simulink model "controller"  (R2023b)
settings: Solver=FixedStepDiscrete  StartTime=0.0  StopTime=inf  FixedStep=1/100  RelTol=1e-3
model workspace (MAT data in the model file):
  dt = Simulink.Parameter
  dt.Value = 0.0025
  dt.DataType = 'auto'
  dt.Complexity = 'real'
  dt.Dimensions = [1 1]
libraries: slpidlib x3
settings Model: Creator=asd  LastModifiedBy=asd
settings SolverCC: InsertRTBMode=Always
settings DataIOCC: ExternalInput=dt  InitialState=[dt]
settings OptimizationCC: DefaultParameterBehavior=Inlined  DefaultUnderspecifiedDataType=single  EnhancedBackFolding=on  PassReuseOutputArgsAs=Individual arguments  ZeroExternalMemoryAtStartup=off  ZeroInternalMemoryAtStartup=off  OptimizeBlockOrder=speed  DifferentSizesBufferReuse=on  OptimizationCustomize=off  LabelGuidedReuse=on  EfficientTunableParamExpr=on
settings DebuggingCC: ParameterTunabilityLossMsg=error
settings HardwareCC: ProdBitPerPointer=32  ProdBitPerSizeT=32  ProdBitPerPtrDiffT=32  ProdLargestAtomicInteger=Long  ProdLargestAtomicFloat=Double  ProdWordSize=32  ProdHWDeviceType=ARM Compatible->ARM Cortex-M
settings SFSimCC: MATLABDynamicMemAlloc=off
settings RTWCC: Description=Embedded Coder  SystemTargetFile=ert.tlc  GenCodeOnly=on  TemplateMakefile=ert_default_tmf  CustomSourceCode="#pragma GCC diagnostic ignored \"-Wfloat-equal\""  DataTypeReplacement=CDataTypesFixedWidth  TargetLang=C++
settings CodeAppCC: ForceParamTrailComments=on  IgnoreCustomStorageClasses=off  OperatorAnnotations=on  SimulinkDataObjDesc=on  SFDataObjDesc=on  InsertBlockDesc=on
settings ERTTargetCC: TargetLangStandard=C++11 (ISO)  GenerateSampleERTMain=on  CombineSignalStateStructs=on  GroupInternalDataByFunction=on  CodeInterfacePackaging=C++ class  SupportComplex=off  DSAsUniqueAccess=on  ExtModeTransport=2  ExtModeStaticAlloc=on  ExtModeMaxTrigDuration=1000000  ExtModeMexFile=ext_xcp  ExtModeIntrfLevel=Level2 - Open  RootIOFormat=Structure reference  ERTCustomFileTemplate=example_file_process.tlc  MaxIdInt64=INT64_MAX  MinIdInt64=INT64_MIN  MaxIdUint64=UINT64_MAX  MaxIdInt32=INT32_MAX  MinIdInt32=INT32_MIN  MaxIdUint32=UINT32_MAX  MaxIdInt16=INT16_MAX  MinIdInt16=INT16_MIN  MaxIdUint16=UINT16_MAX  MaxIdInt8=INT8_MAX  MinIdInt8=INT8_MIN  MaxIdUint8=UINT8_MAX

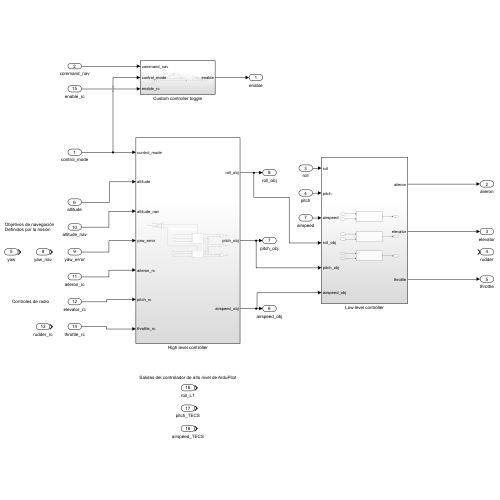
[thumbnail: Simulink's stored preview of the top-level diagram]
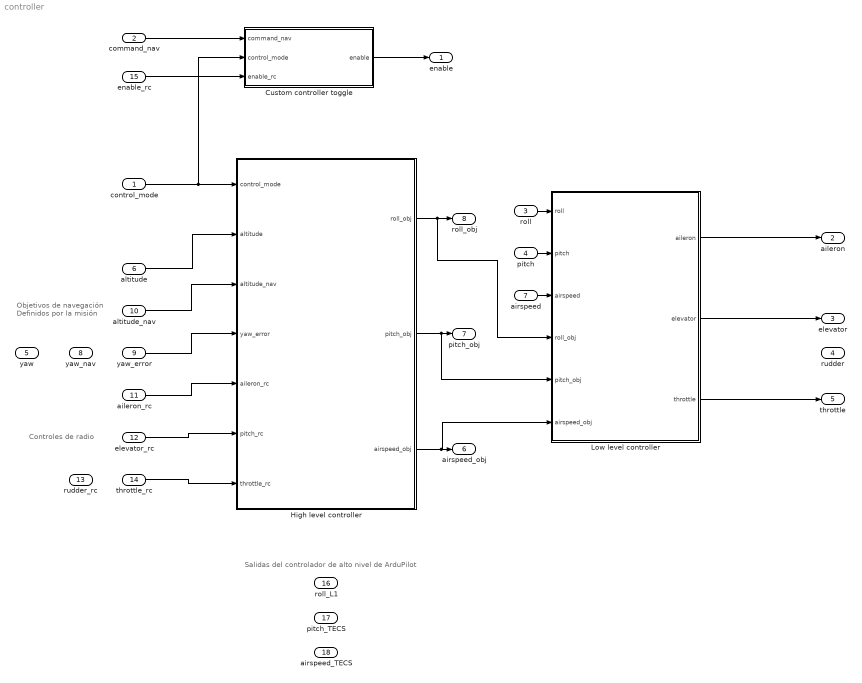
== system controller ==
  note: Controles de radio
  note: Objetivos de navegación
      | Definidos por la misión
  note: Salidas del controlador de alto nivel de ArduPilot
  control_mode : Inport  OutDataTypeStr=single
  command_nav : Inport  Port=2
  roll : Inport  Port=3
  pitch : Inport  Port=4
  yaw : Inport  Port=5
  altitude : Inport  Port=6
  airspeed : Inport  Port=7  OutDataTypeStr=single
  yaw_nav : Inport  Port=8
  yaw_error : Inport  Port=9
  altitude_nav : Inport  Port=10
  aileron_rc : Inport  Port=11
  elevator_rc : Inport  Port=12
  rudder_rc : Inport  Port=13
  throttle_rc : Inport  Port=14  OutDataTypeStr=single
  enable_rc : Inport  Port=15  OutDataTypeStr=boolean
  roll_L1 : Inport  Port=16
  pitch_TECS : Inport  Port=17
  airspeed_TECS : Inport  Port=18
  Custom controller toggle : Subsystem
  High level controller : Subsystem
  Low level controller : Subsystem
  enable : Outport  OutDataTypeStr=boolean
  aileron : Outport  Port=2
  elevator : Outport  Port=3
  rudder : Outport  Port=4
  throttle : Outport  Port=5  OutDataTypeStr=single
  airspeed_obj : Outport  Port=6  OutDataTypeStr=single
  pitch_obj : Outport  Port=7
  roll_obj : Outport  Port=8
  wires:
  control_mode/1 -> Custom controller toggle/2(control_mode), High level controller/1(control_mode)
  altitude/1 -> High level controller/2(altitude)
  altitude_nav/1 -> High level controller/3(altitude_nav)
  yaw_error/1 -> High level controller/4(yaw_error)
  aileron_rc/1 -> High level controller/5(aileron_rc)
  elevator_rc/1 -> High level controller/6(pitch_rc)
  throttle_rc/1 -> High level controller/7(throttle_rc)
  High level controller/1(roll_obj) -> roll_obj/1, Low level controller/4(roll_obj)
  roll/1 -> Low level controller/1(roll)
  High level controller/2(pitch_obj) -> pitch_obj/1, Low level controller/5(pitch_obj)
  pitch/1 -> Low level controller/2(pitch)
  High level controller/3(airspeed_obj) -> Low level controller/6(airspeed_obj), airspeed_obj/1
  Low level controller/1(aileron) -> aileron/1
  Low level controller/2(elevator) -> elevator/1
  Low level controller/3(throttle) -> throttle/1
  airspeed/1 -> Low level controller/3(airspeed)
  command_nav/1 -> Custom controller toggle/1(command_nav)
  Custom controller toggle/1(enable) -> enable/1
  enable_rc/1 -> Custom controller toggle/3(enable_rc)

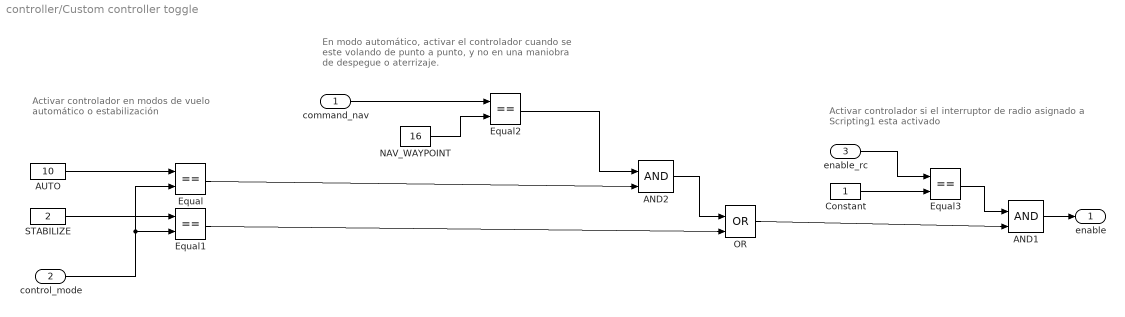
== system controller/Custom controller toggle ==
  note: Activar controlador si el interruptor de radio asignado
      | a Scripting1 esta activado
  note: En modo automático, activar el controlador cuando
      | se este volando de punto a punto, y no en una
      | maniobra de despegue o aterrizaje.
  note: Activar controlador en modos de vuelo
      | automático o estabilización
  command_nav : Inport
  control_mode : Inport  Port=2
  enable_rc : Inport  Port=3  OutDataTypeStr=boolean
  AND1 : Logic  IconShape=distinctive  AllPortsSameDT=off  OutDataTypeStr=boolean
  AND2 : Logic  IconShape=distinctive  AllPortsSameDT=off  OutDataTypeStr=boolean
  AUTO : Constant  Value=10  OutDataTypeStr=single
  Constant : Constant  OutDataTypeStr=boolean
  Equal{,1..3} (4 alike) : RelationalOperator  Operator===  OutDataTypeStr=boolean  RndMeth=Simplest  InputSameDT=off
  NAV_WAYPOINT : Constant  Value=16  OutDataTypeStr=single
  OR : Logic  Operator=OR  IconShape=distinctive  AllPortsSameDT=off  OutDataTypeStr=boolean
  STABILIZE : Constant  Value=2  OutDataTypeStr=single
  enable : Outport
  wires:
  Equal1/1 -> OR/2
  control_mode/1 -> Equal/2, Equal1/2
  STABILIZE/1 -> Equal1/1
  AUTO/1 -> Equal/1
  NAV_WAYPOINT/1 -> Equal2/2
  command_nav/1 -> Equal2/1
  AND1/1 -> enable/1
  Constant/1 -> Equal3/2
  enable_rc/1 -> Equal3/1
  Equal3/1 -> AND1/1
  Equal2/1 -> AND2/1
  Equal/1 -> AND2/2
  AND2/1 -> OR/1
  OR/1 -> AND1/2

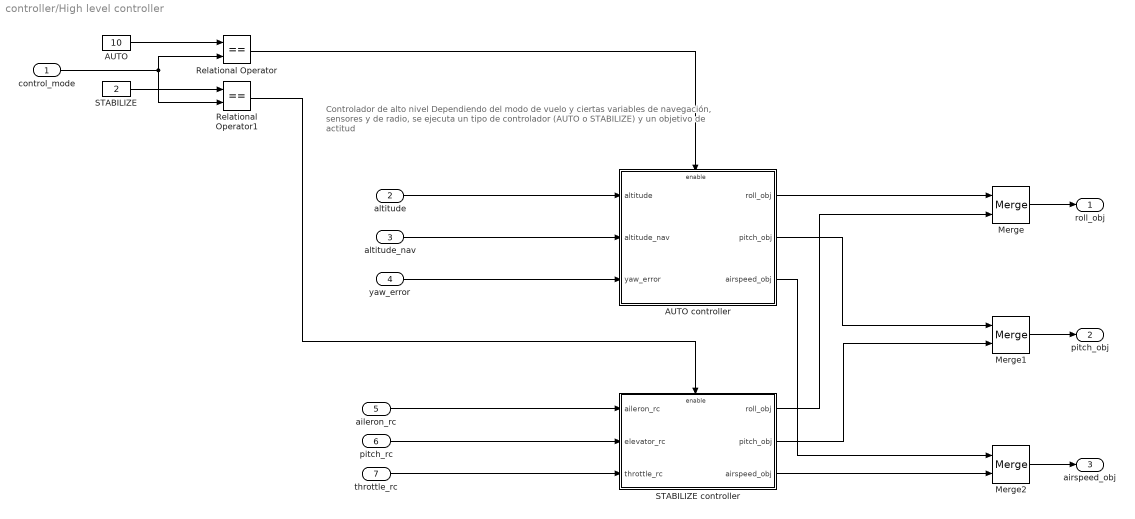
== system controller/High level controller ==
  note: Controlador de alto nivel
      | Dependiendo del modo de vuelo y ciertas variables de navegación, sensores y de radio,
      | se ejecuta un tipo de controlador (AUTO o STABILIZE) y un objetivo de actitud
  control_mode : Inport
  altitude : Inport  Port=2
  altitude_nav : Inport  Port=3
  yaw_error : Inport  Port=4
  aileron_rc : Inport  Port=5
  pitch_rc : Inport  Port=6
  throttle_rc : Inport  Port=7
  AUTO : Constant  Value=10
  AUTO controller : Subsystem
  Merge : Merge
  Merge1 : Merge
  Merge2 : Merge
  Relational Operator : RelationalOperator  Operator===  OutDataTypeStr=boolean  RndMeth=Simplest  InputSameDT=off
  Relational Operator1 : RelationalOperator  Operator===  OutDataTypeStr=boolean  RndMeth=Simplest  InputSameDT=off
  STABILIZE : Constant  Value=2
  STABILIZE controller : Subsystem
  roll_obj : Outport
  pitch_obj : Outport  Port=2
  airspeed_obj : Outport  Port=3
  wires:
  AUTO/1 -> Relational Operator/1
  Merge2/1 -> airspeed_obj/1
  STABILIZE/1 -> Relational Operator1/1
  control_mode/1 -> Relational Operator1/2, Relational Operator/2
  Relational Operator/1 -> AUTO controller/Enable
  pitch_rc/1 -> STABILIZE controller/2(elevator_rc)
  Relational Operator1/1 -> STABILIZE controller/Enable
  altitude_nav/1 -> AUTO controller/2(altitude_nav)
  yaw_error/1 -> AUTO controller/3(yaw_error)
  altitude/1 -> AUTO controller/1(altitude)
  Merge/1 -> roll_obj/1
  throttle_rc/1 -> STABILIZE controller/3(throttle_rc)
  aileron_rc/1 -> STABILIZE controller/1(aileron_rc)
  Merge1/1 -> pitch_obj/1
  AUTO controller/1(roll_obj) -> Merge/1
  STABILIZE controller/1(roll_obj) -> Merge/2
  AUTO controller/2(pitch_obj) -> Merge1/1
  STABILIZE controller/2(pitch_obj) -> Merge1/2
  STABILIZE controller/3(airspeed_obj) -> Merge2/2
  AUTO controller/3(airspeed_obj) -> Merge2/1

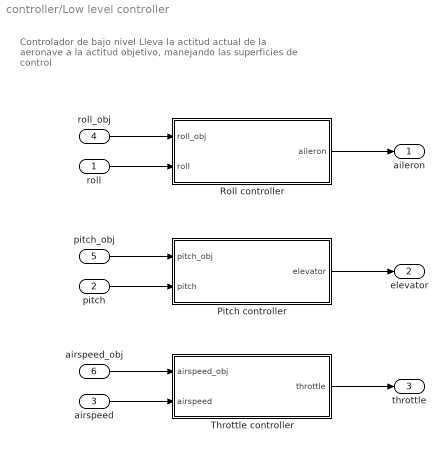
== system controller/Low level controller ==
  note: Controlador de bajo nivel
      | Lleva la actitud actual de la aeronave a la actitud objetivo,
      | manejando las superficies de control
  roll : Inport
  pitch : Inport  Port=2
  airspeed : Inport  Port=3
  roll_obj : Inport  Port=4
  pitch_obj : Inport  Port=5
  airspeed_obj : Inport  Port=6
  Pitch controller : Subsystem
  Roll controller : Subsystem
  Throttle controller : Subsystem
  aileron : Outport
  elevator : Outport  Port=2
  throttle : Outport  Port=3
  wires:
  Pitch controller/1(elevator) -> elevator/1
  Throttle controller/1(throttle) -> throttle/1
  roll/1 -> Roll controller/2(roll)
  pitch/1 -> Pitch controller/2(pitch)
  pitch_obj/1 -> Pitch controller/1(pitch_obj)
  Roll controller/1(aileron) -> aileron/1
  roll_obj/1 -> Roll controller/1(roll_obj)
  airspeed_obj/1 -> Throttle controller/1(airspeed_obj)
  airspeed/1 -> Throttle controller/2(airspeed)

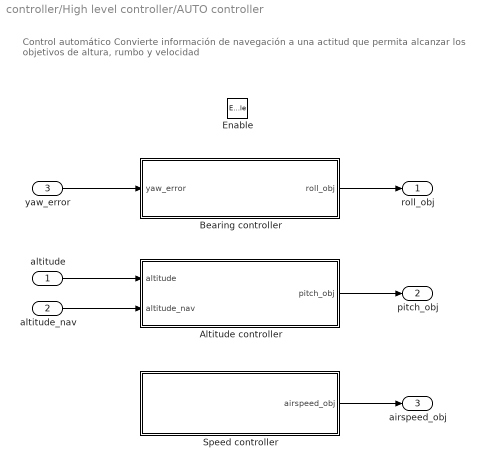
== system controller/High level controller/AUTO controller ==
  note: Control automático
      | Convierte información de navegación a una actitud que permita alcanzar los objetivos de altura, rumbo y velocidad
  altitude : Inport
  altitude_nav : Inport  Port=2
  yaw_error : Inport  Port=3
  Enable : EnablePort
  Altitude controller : Subsystem
  Bearing controller : Subsystem
  Speed controller : Subsystem
  roll_obj : Outport
  pitch_obj : Outport  Port=2
  airspeed_obj : Outport  Port=3
  wires:
  yaw_error/1 -> Bearing controller/1(yaw_error)
  altitude_nav/1 -> Altitude controller/2(altitude_nav)
  altitude/1 -> Altitude controller/1(altitude)
  Speed controller/1(airspeed_obj) -> airspeed_obj/1
  Bearing controller/1(roll_obj) -> roll_obj/1
  Altitude controller/1(pitch_obj) -> pitch_obj/1

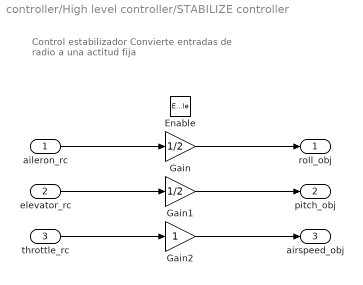
== system controller/High level controller/STABILIZE controller ==
  note: Control estabilizador
      | Convierte entradas de radio a una actitud fija
  aileron_rc : Inport
  elevator_rc : Inport  Port=2
  throttle_rc : Inport  Port=3
  Enable : EnablePort
  Gain : Gain  Gain=1/2
  Gain1 : Gain  Gain=1/2
  Gain2 : Gain
  roll_obj : Outport
  pitch_obj : Outport  Port=2
  airspeed_obj : Outport  Port=3
  wires:
  elevator_rc/1 -> Gain1/1
  aileron_rc/1 -> Gain/1
  Gain2/1 -> airspeed_obj/1
  throttle_rc/1 -> Gain2/1
  Gain1/1 -> pitch_obj/1
  Gain/1 -> roll_obj/1

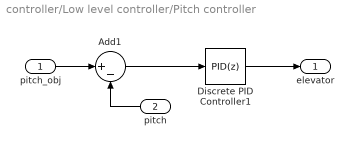
== system controller/Low level controller/Pitch controller ==
  pitch_obj : Inport
  pitch : Inport  Port=2
  Add1 : Sum  Inputs=|+-
  Discrete PID Controller1 : slpidlib/PID Controller  Controller=PID  Form=Parallel  TimeDomain=Discrete-time  UseExternalTs=off  SampleTime=-1  IntegratorMethod=Forward Euler  FilterMethod=Forward Euler  ControllerParametersSource=internal  P=1  I=0.1  UseKiTs=off  D=0.1  N=100  UseFilter=on  TunerSelectOption=Transfer Function Based (PID Tuner App)  InitialConditionSource=internal  InitialConditionForIntegrator=0  InitialConditionForFilter=0  DifferentiatorICPrevScaledInput=0  ExternalReset=none  TrackingMode=off  Kt=1  LimitOutput=off  SatLimitsSource=internal  UpperSaturationLimit=inf  LowerSaturationLimit=-inf  LinearizeAsGain=off  AntiWindupMode=none  Kb=1  LimitIntegrator=off  UpperIntegratorSaturationLimit=inf  LowerIntegratorSaturationLimit=-inf  POutMin=[]  POutMax=[]  IOutMin=[]  IOutMax=[]  DOutMin=[]  DOutMax=[]  NOutMin=[]  NOutMax=[]  SumOutMin=[]  SumOutMax=[]  SaturationOutMin=[]  SaturationOutMax=[]  PParamMin=[]  PParamMax=[]  IParamMin=[]  IParamMax=[]  DParamMin=[]  DParamMax=[]  NParamMin=[]  NParamMax=[]  KbParamMin=[]  KbParamMax=[]  KtParamMin=[]  KtParamMax=[]  KbOutMin=[]  KbOutMax=[]  KtOutMin=[]  KtOutMax=[]  IntegratorOutMin=[]  IntegratorOutMax=[]  FilterOutMin=[]  FilterOutMax=[]  SumI1OutMin=[]  SumI1OutMax=[]  SumI2OutMin=[]  SumI2OutMax=[]  SumI3OutMin=[]  SumI3OutMax=[]  SumI4OutMin=[]  SumI4OutMax=[]  SumDOutMin=[]  SumDOutMax=[]  DifferentiatorOutMin=[]  DifferentiatorOutMax=[]  FilterDiffOutCoefMin=[]  FilterDiffOutCoefMax=[]  ReciprocalOutMin=[]  ReciprocalOutMax=[]  SumDenOutMin=[]  SumDenOutMax=[]  SumNumOutMin=[]  SumNumOutMax=[]  DivideOutMin=[]  DivideOutMax=[]  UdiffTsProdOutMin=[]  UdiffTsProdOutMax=[]  NTsProdOutMin=[]  NTsProdOutMax=[]  UintegralTsProdOutMin=[]  UintegralTsProdOutMax=[]  UngainTsProdOutMin=[]  UngainTsProdOutMax=[]  ClampingZeroOutDataTypeStr=Inherit: Inherit via back propagation  ClampingZeroOutMin=[]  ClampingZeroOutMax=[]  FilterDenConstantOutDataTypeStr=Inherit: Inherit via back propagation  FilterDenConstantOutMin=[]  FilterDenConstantOutMax=[]  PCopyOutDataTypeStr=Inherit: Inherit via back propagation  PCopyOutMin=[]  PCopyOutMax=[]  NCopyOutDataTypeStr=Inherit: Inherit via back propagation  NCopyOutMin=[]  NCopyOutMax=[]  IntegratorContinuousStateAttributes=''  IntegratorStateMustResolveToSignalObject=off  IntegratorRTWStateStorageClass=Auto  FilterContinuousStateAttributes=''  FilterStateMustResolveToSignalObject=off  FilterRTWStateStorageClass=Auto  ParallelPVariant=InternalParameters  IdealPVariant=Disabled  IVariant=InternalParameters  DVariant=InternalParameters  IntegratorVariant=Discrete  SatVariant=Disabled  AWVariant=Passthrough  PCopyVariant=Disabled  TRVariant=Disabled  FdbkBlocksVariant=Forward  IdealPFdbkVariant=Disabled  SatFdbkVariant=Disabled  DerivativeFilterVariant=ForwardEulerFilter  NVariant=InternalParameters  NCopyVariant=Disabled  FilterICVariant=InternalICsFilter  IntegratorICVariant=InternalICs  ExternalResetVariant=Disabled  TRSumVariant=Passthrough  SumFdbkVariant=Disabled  SumVariant=Sum_PID  TsampFilterVariant=InternalTs  TsampNgainVariant=Passthrough  TsampIntegralVariant=Disabled_SignalSpec  ExternalSaturationOutDataTypeStr=Inherit: Same as second input
      settings: LibrarySourceBlock=simulink/Discrete/Discrete PID Controller
  elevator : Outport
  wires:
  pitch_obj/1 -> Add1/1
  Add1/1 -> Discrete PID Controller1/1
  Discrete PID Controller1/1 -> elevator/1
  pitch/1 -> Add1/2

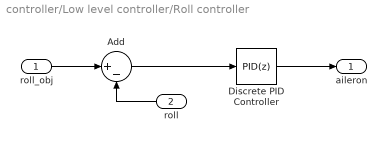
== system controller/Low level controller/Roll controller ==
  roll_obj : Inport
  roll : Inport  Port=2
  Add : Sum  Inputs=|+-
  Discrete PID Controller : slpidlib/PID Controller  Controller=PID  Form=Parallel  TimeDomain=Discrete-time  UseExternalTs=off  SampleTime=-1  IntegratorMethod=Forward Euler  FilterMethod=Forward Euler  ControllerParametersSource=internal  P=1  I=0  UseKiTs=off  D=0.5  N=100  UseFilter=on  TunerSelectOption=Transfer Function Based (PID Tuner App)  InitialConditionSource=internal  InitialConditionForIntegrator=0  InitialConditionForFilter=0  DifferentiatorICPrevScaledInput=0  ExternalReset=none  TrackingMode=off  Kt=1  LimitOutput=off  SatLimitsSource=internal  UpperSaturationLimit=inf  LowerSaturationLimit=-inf  LinearizeAsGain=off  AntiWindupMode=none  Kb=1  LimitIntegrator=off  UpperIntegratorSaturationLimit=inf  LowerIntegratorSaturationLimit=-inf  POutMin=[]  POutMax=[]  IOutMin=[]  IOutMax=[]  DOutMin=[]  DOutMax=[]  NOutMin=[]  NOutMax=[]  SumOutMin=[]  SumOutMax=[]  SaturationOutMin=[]  SaturationOutMax=[]  PParamMin=[]  PParamMax=[]  IParamMin=[]  IParamMax=[]  DParamMin=[]  DParamMax=[]  NParamMin=[]  NParamMax=[]  KbParamMin=[]  KbParamMax=[]  KtParamMin=[]  KtParamMax=[]  KbOutMin=[]  KbOutMax=[]  KtOutMin=[]  KtOutMax=[]  IntegratorOutMin=[]  IntegratorOutMax=[]  FilterOutMin=[]  FilterOutMax=[]  SumI1OutMin=[]  SumI1OutMax=[]  SumI2OutMin=[]  SumI2OutMax=[]  SumI3OutMin=[]  SumI3OutMax=[]  SumI4OutMin=[]  SumI4OutMax=[]  SumDOutMin=[]  SumDOutMax=[]  DifferentiatorOutMin=[]  DifferentiatorOutMax=[]  FilterDiffOutCoefMin=[]  FilterDiffOutCoefMax=[]  ReciprocalOutMin=[]  ReciprocalOutMax=[]  SumDenOutMin=[]  SumDenOutMax=[]  SumNumOutMin=[]  SumNumOutMax=[]  DivideOutMin=[]  DivideOutMax=[]  UdiffTsProdOutMin=[]  UdiffTsProdOutMax=[]  NTsProdOutMin=[]  NTsProdOutMax=[]  UintegralTsProdOutMin=[]  UintegralTsProdOutMax=[]  UngainTsProdOutMin=[]  UngainTsProdOutMax=[]  ClampingZeroOutDataTypeStr=Inherit: Inherit via back propagation  ClampingZeroOutMin=[]  ClampingZeroOutMax=[]  FilterDenConstantOutDataTypeStr=Inherit: Inherit via back propagation  FilterDenConstantOutMin=[]  FilterDenConstantOutMax=[]  PCopyOutDataTypeStr=Inherit: Inherit via back propagation  PCopyOutMin=[]  PCopyOutMax=[]  NCopyOutDataTypeStr=Inherit: Inherit via back propagation  NCopyOutMin=[]  NCopyOutMax=[]  IntegratorContinuousStateAttributes=''  IntegratorStateMustResolveToSignalObject=off  IntegratorRTWStateStorageClass=Auto  FilterContinuousStateAttributes=''  FilterStateMustResolveToSignalObject=off  FilterRTWStateStorageClass=Auto  ParallelPVariant=InternalParameters  IdealPVariant=Disabled  IVariant=InternalParameters  DVariant=InternalParameters  IntegratorVariant=Discrete  SatVariant=Disabled  AWVariant=Passthrough  PCopyVariant=Disabled  TRVariant=Disabled  FdbkBlocksVariant=Forward  IdealPFdbkVariant=Disabled  SatFdbkVariant=Disabled  DerivativeFilterVariant=ForwardEulerFilter  NVariant=InternalParameters  NCopyVariant=Disabled  FilterICVariant=InternalICsFilter  IntegratorICVariant=InternalICs  ExternalResetVariant=Disabled  TRSumVariant=Passthrough  SumFdbkVariant=Disabled  SumVariant=Sum_PID  TsampFilterVariant=InternalTs  TsampNgainVariant=Passthrough  TsampIntegralVariant=Disabled_SignalSpec  ExternalSaturationOutDataTypeStr=Inherit: Same as second input
      settings: LibrarySourceBlock=simulink/Discrete/Discrete PID Controller
  aileron : Outport
  wires:
  Add/1 -> Discrete PID Controller/1
  roll/1 -> Add/2
  Discrete PID Controller/1 -> aileron/1
  roll_obj/1 -> Add/1

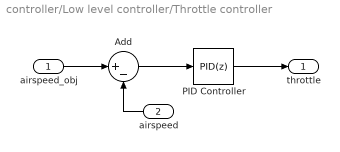
== system controller/Low level controller/Throttle controller ==
  airspeed_obj : Inport
  airspeed : Inport  Port=2
  Add : Sum  Inputs=|+-
  PID Controller : slpidlib/PID Controller  Controller=PID  Form=Parallel  TimeDomain=Discrete-time  UseExternalTs=off  SampleTime=-1  IntegratorMethod=Forward Euler  FilterMethod=Forward Euler  ControllerParametersSource=internal  P=5  I=1  UseKiTs=off  D=1  N=100  UseFilter=on  TunerSelectOption=Transfer Function Based (PID Tuner App)  InitialConditionSource=internal  InitialConditionForIntegrator=0  InitialConditionForFilter=0  DifferentiatorICPrevScaledInput=0  ExternalReset=none  TrackingMode=off  Kt=1  LimitOutput=off  SatLimitsSource=internal  UpperSaturationLimit=inf  LowerSaturationLimit=-inf  LinearizeAsGain=on  AntiWindupMode=none  Kb=1  LimitIntegrator=off  UpperIntegratorSaturationLimit=inf  LowerIntegratorSaturationLimit=-inf  POutMin=[]  POutMax=[]  IOutMin=[]  IOutMax=[]  DOutMin=[]  DOutMax=[]  NOutMin=[]  NOutMax=[]  SumOutMin=[]  SumOutMax=[]  SaturationOutMin=[]  SaturationOutMax=[]  PParamMin=[]  PParamMax=[]  IParamMin=[]  IParamMax=[]  DParamMin=[]  DParamMax=[]  NParamMin=[]  NParamMax=[]  KbParamMin=[]  KbParamMax=[]  KtParamMin=[]  KtParamMax=[]  KbOutMin=[]  KbOutMax=[]  KtOutMin=[]  KtOutMax=[]  IntegratorOutMin=[]  IntegratorOutMax=[]  FilterOutMin=[]  FilterOutMax=[]  SumI1OutMin=[]  SumI1OutMax=[]  SumI2OutMin=[]  SumI2OutMax=[]  SumI3OutMin=[]  SumI3OutMax=[]  SumI4OutMin=[]  SumI4OutMax=[]  SumDOutMin=[]  SumDOutMax=[]  DifferentiatorOutMin=[]  DifferentiatorOutMax=[]  FilterDiffOutCoefMin=[]  FilterDiffOutCoefMax=[]  ReciprocalOutMin=[]  ReciprocalOutMax=[]  SumDenOutMin=[]  SumDenOutMax=[]  SumNumOutMin=[]  SumNumOutMax=[]  DivideOutMin=[]  DivideOutMax=[]  UdiffTsProdOutMin=[]  UdiffTsProdOutMax=[]  NTsProdOutMin=[]  NTsProdOutMax=[]  UintegralTsProdOutMin=[]  UintegralTsProdOutMax=[]  UngainTsProdOutMin=[]  UngainTsProdOutMax=[]  ClampingZeroOutDataTypeStr=Inherit: Inherit via back propagation  ClampingZeroOutMin=[]  ClampingZeroOutMax=[]  FilterDenConstantOutDataTypeStr=Inherit: Inherit via back propagation  FilterDenConstantOutMin=[]  FilterDenConstantOutMax=[]  PCopyOutDataTypeStr=Inherit: Inherit via back propagation  PCopyOutMin=[]  PCopyOutMax=[]  NCopyOutDataTypeStr=Inherit: Inherit via back propagation  NCopyOutMin=[]  NCopyOutMax=[]  IntegratorContinuousStateAttributes=''  IntegratorStateMustResolveToSignalObject=off  IntegratorRTWStateStorageClass=Auto  FilterContinuousStateAttributes=''  FilterStateMustResolveToSignalObject=off  FilterRTWStateStorageClass=Auto  ParallelPVariant=InternalParameters  IdealPVariant=Disabled  IVariant=InternalParameters  DVariant=InternalParameters  IntegratorVariant=Discrete  SatVariant=Disabled  AWVariant=Passthrough  PCopyVariant=Disabled  TRVariant=Disabled  FdbkBlocksVariant=Forward  IdealPFdbkVariant=Disabled  SatFdbkVariant=Disabled  DerivativeFilterVariant=ForwardEulerFilter  NVariant=InternalParameters  NCopyVariant=Disabled  FilterICVariant=InternalICsFilter  IntegratorICVariant=InternalICs  ExternalResetVariant=Disabled  TRSumVariant=Passthrough  SumFdbkVariant=Disabled  SumVariant=Sum_PID  TsampFilterVariant=InternalTs  TsampNgainVariant=Passthrough  TsampIntegralVariant=Disabled_SignalSpec  ExternalSaturationOutDataTypeStr=Inherit: Same as second input
  throttle : Outport
  wires:
  airspeed_obj/1 -> Add/1
  airspeed/1 -> Add/2
  PID Controller/1 -> throttle/1
  Add/1 -> PID Controller/1

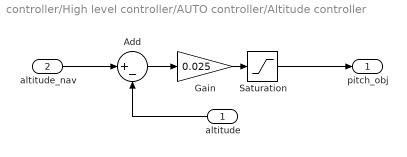
== system controller/High level controller/AUTO controller/Altitude controller ==
  altitude : Inport
  altitude_nav : Inport  Port=2
  Add : Sum  Inputs=|+-
  Gain : Gain  Gain=0.025
  Saturation : Saturate  UpperLimit=pi/6  LowerLimit=-pi/6
  pitch_obj : Outport
  wires:
  altitude_nav/1 -> Add/1
  Add/1 -> Gain/1
  Saturation/1 -> pitch_obj/1
  altitude/1 -> Add/2
  Gain/1 -> Saturation/1

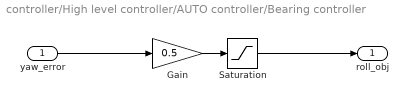
== system controller/High level controller/AUTO controller/Bearing controller ==
  yaw_error : Inport
  Gain : Gain  Gain=0.5
  Saturation : Saturate  UpperLimit=pi/4  LowerLimit=-pi/4
  roll_obj : Outport
  wires:
  yaw_error/1 -> Gain/1
  Saturation/1 -> roll_obj/1
  Gain/1 -> Saturation/1

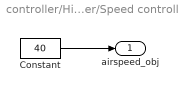
== system controller/High level controller/AUTO controller/Speed controller ==
  Constant : Constant  Value=40  OutDataTypeStr=single
  airspeed_obj : Outport
  wires:
  Constant/1 -> airspeed_obj/1
